simulink model "aircraft_BO_sim"  (R2021b)
settings: Solver=ode45  StartTime=0.0  StopTime=50  RelTol=1e-3  EnableMultiTasking=on
values from neighbouring files (symbols this model uses):
  CD_0 = 0.02    [aircraft_data.m]
  CD_2 = 0.0335    [aircraft_data.m]
  CG = [0 0 0]'    [aircraft_data.m]
  chord = 4.29    [aircraft_data.m]
  CL_0 = 0.11    [aircraft_data.m]
  CL_alpha = 5.5    [aircraft_data.m]
  CL_alphadot = 2.7    [aircraft_data.m]
  Cl_beta = -0.03    [aircraft_data.m]
  Cl_da = -0.07    [aircraft_data.m]
  CL_de = 0.32    [aircraft_data.m]
  Cl_dr = 0.02    [aircraft_data.m]
  CL_dths = -0.32    [aircraft_data.m]
  Cl_p = -0.5    [aircraft_data.m]
  CL_q = 3.3    [aircraft_data.m]
  Cl_r_0 = 0.15    [aircraft_data.m]
  Cl_r_alpha = 0.035    [aircraft_data.m]
  Cm_0 = 0.02    [aircraft_data.m]
  Cm_alpha = -1.5    [aircraft_data.m]
  Cm_alphadot = -12    [aircraft_data.m]
  Cm_de = -1.2    [aircraft_data.m]
  Cm_dths = 1.2    [aircraft_data.m]
  Cm_q = -12    [aircraft_data.m]
  Cn_beta_0 = 0.2    [aircraft_data.m]
  Cn_beta_alpha = -0.0195    [aircraft_data.m]
  Cn_da = -0.03    [aircraft_data.m]
  Cn_dr = -0.09    [aircraft_data.m]
  Cn_p_0 = -0.025    [aircraft_data.m]
  Cn_p_alpha = -0.035    [aircraft_data.m]
  Cn_r = -0.18    [aircraft_data.m]
  CY_beta = -1.42    [aircraft_data.m]
  CY_da = 0.0    (= 0)    [aircraft_data.m]
  CY_dr = 0.05    [aircraft_data.m]
  CY_p = 0.0    (= 0)    [aircraft_data.m]
  CY_r = 0.0    (= 0)    [aircraft_data.m]
  dths_e = x(2)    [trimmed_equations.m]
  em = 1*pi/180    (= 0.0174532925199)    [aircraft_data.m]
  g0 = 9.80665    [aircraft_data.m]
  gamma = 1.4    [aircraft_data.m]
  h0 = 0    [aircraft_data.m]
  h_strat = 20000    [aircraft_data.m]
  h_trop = 11000    [aircraft_data.m]
  Ib = [ Ixx 0   -Ixz ... (first row only)    [aircraft_data.m]
  LEngLoc = [xm -ym zm]'    [aircraft_data.m]
  mass = 57837.5    [aircraft_data.m]
  P0 = 101325    [aircraft_data.m]
  R = 287.0531    [aircraft_data.m]
  REngLoc = [xm  ym zm]'    [aircraft_data.m]
  rho0 = 1.225    [aircraft_data.m]
  T0 = 288.15    [aircraft_data.m]
  Th = -0.0065    [aircraft_data.m]
  wingarea = 122.6    [aircraft_data.m]
  wingspan = 34.10    (= 34.1)    [aircraft_data.m]
undefined symbols (not defined in the file or in its folder): da_e, de_e, dr_e, dth_e, Euler_e, Newton, Omegab_e, Po_e, Raphson, Vb_e
settings Model: Creator=David  LastModifiedBy=dsaussie
settings SolverCC: AlgebraicLoopSolver=TrustRegion
settings DataIOCC: LimitDataPoints=on  SaveFormat=Array  ReturnWorkspaceOutputs=off
settings OptimizationCC: BlockReduction=off  BooleanDataType=off  LifeSpan=inf
settings DebuggingCC: AlgebraicLoopMsg=none  SaveWithParameterizedLinksMsg=none  UnderspecifiedInitializationDetection=Classic  MergeDetectMultiDrivingBlocksExec=none  SignalResolutionControl=TryResolveAllWithWarning  SFUnexpectedBacktrackingDiag=warning  SFNoUnconditionalDefaultTransitionDiag=warning  SFExecutionAtInitializationDiag=none  SFMachineParentedDataDiag=warning  ArithmeticOperatorsInVariantConditions=warning
settings HardwareCC: ProdBitPerPointer=32  ProdBitPerSizeT=32  ProdBitPerPtrDiffT=32  ProdLargestAtomicFloat=None  ProdIntDivRoundTo=Undefined  ProdEndianess=Unspecified  ProdWordSize=32  ProdHWDeviceType=32-bit Generic  TargetUnknown=on
settings ModelReferenceCC: PropagateSignalLabelsOutOfModel=off
settings SFSimCC: SimUseLocalCustomCode=off  CustomCodeUndefinedFunction=UseInterfaceOnly
settings RTWCC: RTWUseLocalCustomCode=off
settings CodeAppCC: StateflowObjectComments=on
settings GRTTargetCC: TargetLangStandard=C89/C90 (ANSI)
settings ConfigComp: CovMetricSettings=dw  CovSaveCumulativeToWorkspaceVar=on  CovSaveSingleToWorkspaceVar=on  CovExternalEMLEnable=off  CovSFcnEnable=off

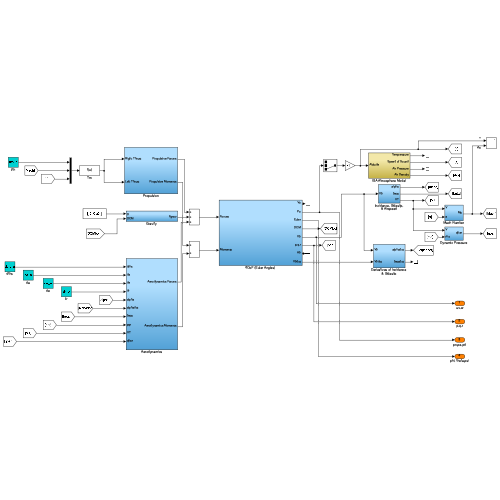
[thumbnail: Simulink's stored preview of the top-level diagram]
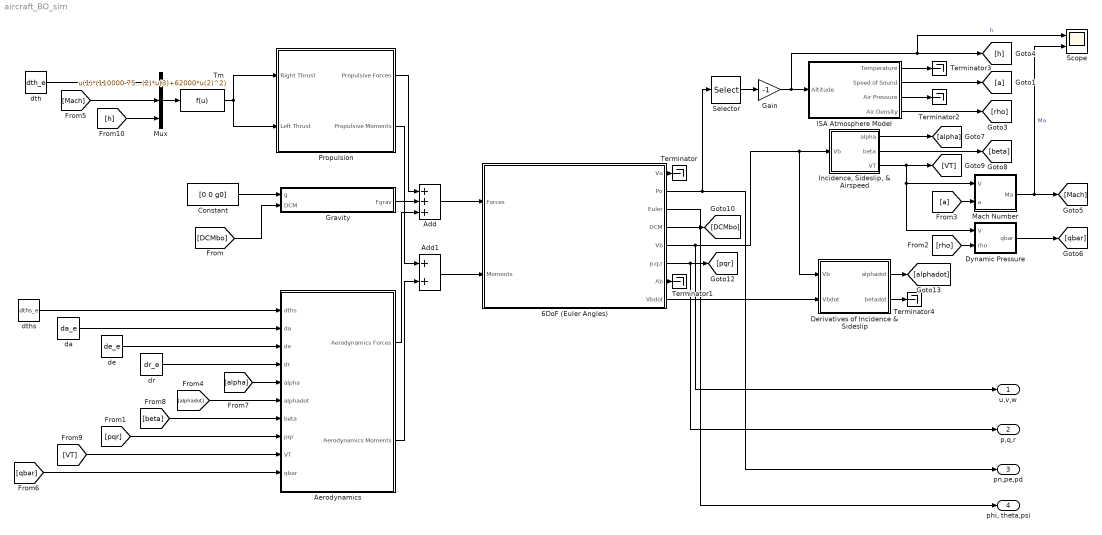
== system aircraft_BO_sim ==
  6DoF (Euler Angles) : Subsystem
  Add : Sum  Inputs=+++
  Add1 : Sum
  Aerodynamics : Subsystem
  Constant : Constant  Value=[0 0 g0]
  Derivatives of Incidence & Sideslip : Subsystem
  Dynamic Pressure : Subsystem
  Gain : Gain  Gain=-1
  "Gravity " : Subsystem
  ISA Atmosphere Model : Subsystem
  "Incidence, Sideslip, & Airspeed" : Subsystem
  Mach Number : Subsystem
  Mux : Mux  Inputs=3
  Propulsion : Subsystem
  Scope : Scope  NumInputPorts=2
  Selector : Selector  InputPortWidth=3  IndexOptions=Index vector (dialog)  Indices=[3]  OutputSizes=1
  Terminator{,1..4} (5 alike) : Terminator
  Tm : Fcn  Expr=u(1)*(110000-75000*u(2)-7.5*u(3)+2*u(2)*u(3)+62000*u(2)^2)
  da : Constant  Value=da_e
  de : Constant  Value=de_e
  dr : Constant  Value=dr_e
  dth : Constant  Value=dth_e
  dths : Constant  Value=dths_e
  u,v,w : Outport
  p,q,r : Outport  Port=2
  pn,pe,pd : Outport  Port=3
  "phi, theta,psi" : Outport  Port=4
  wires:
  Selector/1 -> Gain/1
  ISA Atmosphere Model/1(Temperature) -> Terminator3/1
  ISA Atmosphere Model/2(Speed of Sound) -> [a]
  ISA Atmosphere Model/3(Air Pressure) -> Terminator2/1
  ISA Atmosphere Model/4(Air Density) -> [rho]
  Mach Number/1(Ma) -> Scope/2, [Mach]  "Ma"
  [a] -> Mach Number/2(a)
  [rho] -> Dynamic Pressure/2(rho)
  Dynamic Pressure/1(qbar) -> [qbar]
  "Incidence, Sideslip, & Airspeed"/3(VT) -> Dynamic Pressure/1(V), Mach Number/1(V), [VT]
  "Incidence, Sideslip, & Airspeed"/1(alpha) -> [alpha]
  "Incidence, Sideslip, & Airspeed"/2(beta) -> [beta]
  6DoF (Euler Angles)/4(DCM) -> [DCMbo]
  Propulsion/1(Propulsive Forces) -> Add/1
  Propulsion/2(Propulsive Moments) -> Add1/1
  de/1 -> Aerodynamics/3(de)
  [alpha] -> Aerodynamics/5(alpha)
  [beta] -> Aerodynamics/7(beta)
  [qbar] -> Aerodynamics/10(qbar)
  [VT] -> Aerodynamics/9(VT)
  Aerodynamics/1(Aerodynamics Forces) -> Add/3
  Aerodynamics/2(Aerodynamics Moments) -> Add1/2
  [pqr] -> Aerodynamics/8(pqr)
  [DCMbo] -> "Gravity "/2(DCM)
  Constant/1 -> "Gravity "/1(g)
  "Gravity "/1(Fgrav) -> Add/2
  dth/1 -> Mux/1
  Add/1 -> 6DoF (Euler Angles)/1(Forces)
  Add1/1 -> 6DoF (Euler Angles)/2(Moments)
  6DoF (Euler Angles)/2(Po) -> pn,pe,pd/1, Selector/1
  6DoF (Euler Angles)/3(Euler) -> "phi, theta,psi"/1
  6DoF (Euler Angles)/6(p,q,r) -> p,q,r/1, [pqr]
  6DoF (Euler Angles)/5(Vb) -> u,v,w/1, Derivatives of Incidence & Sideslip/1(Vb), "Incidence, Sideslip, & Airspeed"/1(Vb)
  dr/1 -> Aerodynamics/4(dr)
  da/1 -> Aerodynamics/2(da)
  6DoF (Euler Angles)/8(Vbdot) -> Derivatives of Incidence & Sideslip/2(Vbdot)
  Derivatives of Incidence & Sideslip/1(alphadot) -> [alphadot]
  Derivatives of Incidence & Sideslip/2(betadot) -> Terminator4/1
  [alphadot] -> Aerodynamics/6(alphadot)
  Mux/1 -> Tm/1
  6DoF (Euler Angles)/1(Vo) -> Terminator/1
  6DoF (Euler Angles)/7(Ab) -> Terminator1/1
  Gain/1 -> ISA Atmosphere Model/1(Altitude), Scope/1, [h]  "h"
  [Mach] -> Mux/2
  [h] -> Mux/3
  Tm/1 -> Propulsion/1(Right Thrust), Propulsion/2(Left Thrust)
  dths/1 -> Aerodynamics/1(dths)

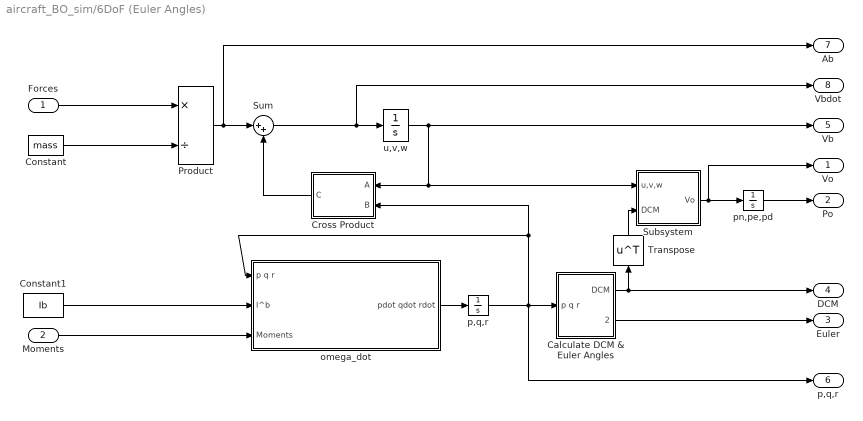
== system aircraft_BO_sim/6DoF (Euler Angles) ==
  Forces : Inport
  Moments : Inport  Port=2
  "Calculate DCM & Euler Angles " : Subsystem
  Constant : Constant  Value=mass  OutDataTypeStr=Inherit: Inherit via back propagation
  Constant1 : Constant  Value=Ib  OutDataTypeStr=Inherit: Inherit via back propagation
  Cross Product : Subsystem
  Product : Product  Inputs=*/  SaturateOnIntegerOverflow=on  OutDataTypeStr=Inherit: Same as first input
  Subsystem : Subsystem
  Sum : Sum  Inputs=|++  SaturateOnIntegerOverflow=on
  Transpose : Math  Operator=transpose  SignedPower=on  SaturateOnIntegerOverflow=on
  omega_dot : Subsystem
  "p,q,r " : Integrator  InitialCondition=Omegab_e
  pn,pe,pd : Integrator  InitialCondition=Po_e
  u,v,w : Integrator  InitialCondition=Vb_e
  Vo : Outport
  Po : Outport  Port=2
  Euler : Outport  Port=3
  DCM : Outport  Port=4
  Vb : Outport  Port=5
  p,q,r : Outport  Port=6
  Ab : Outport  Port=7
  Vbdot : Outport  Port=8
  wires:
  Moments/1 -> omega_dot/3(Moments)
  "p,q,r "/1 -> Cross Product/2(B), omega_dot/1(p q r), p,q,r/1, "Calculate DCM & Euler Angles "/1("p q r ")
  Sum/1 -> Vbdot/1, u,v,w/1
  u,v,w/1 -> Vb/1, Cross Product/1(A), Subsystem/1(u,v,w)
  Subsystem/1(Vo) -> Vo/1, pn,pe,pd/1
  pn,pe,pd/1 -> Po/1
  Forces/1 -> Product/1
  Constant/1 -> Product/2
  Transpose/1 -> Subsystem/2(DCM)
  "Calculate DCM & Euler Angles "/1("DCM ") -> DCM/1, Transpose/1
  Product/1 -> Ab/1, Sum/1
  Cross Product/1(C) -> Sum/2
  "Calculate DCM & Euler Angles "/2(Euler) -> Euler/1
  Constant1/1 -> omega_dot/2(I^b)
  omega_dot/1(pdot qdot rdot) -> "p,q,r "/1

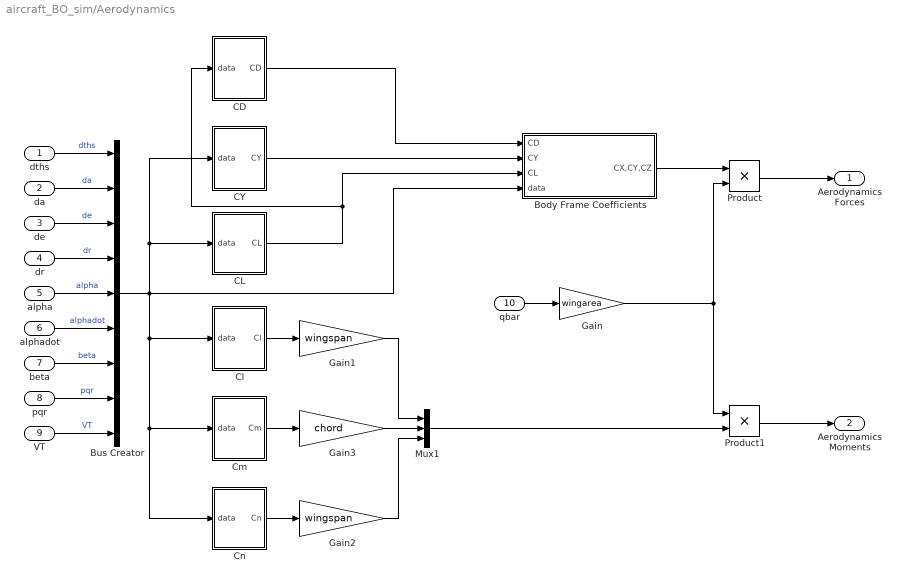
== system aircraft_BO_sim/Aerodynamics ==
  dths : Inport
  da : Inport  Port=2
  de : Inport  Port=3
  dr : Inport  Port=4
  alpha : Inport  Port=5
  alphadot : Inport  Port=6
  beta : Inport  Port=7
  pqr : Inport  Port=8
  VT : Inport  Port=9
  qbar : Inport  Port=10
  Body Frame Coefficients : Subsystem
  Bus Creator : BusCreator  Inputs=9
  CD : Subsystem
  CL : Subsystem
  CY : Subsystem
  Cl : Subsystem
  Cm : Subsystem
  Cn : Subsystem
  Gain : Gain  Gain=wingarea
  Gain1 : Gain  Gain=wingspan
  Gain2 : Gain  Gain=wingspan
  Gain3 : Gain  Gain=chord
  Mux1 : Mux  Inputs=3
  Product : Product  RndMeth=Zero
  Product1 : Product  RndMeth=Zero
  Aerodynamics Forces : Outport
  Aerodynamics Moments : Outport  Port=2
  wires:
  de/1 -> Bus Creator/3  "de"
  da/1 -> Bus Creator/2  "da"
  dr/1 -> Bus Creator/4  "dr"
  alpha/1 -> Bus Creator/5  "alpha"
  beta/1 -> Bus Creator/7  "beta"
  pqr/1 -> Bus Creator/8  "pqr"
  Bus Creator/1 -> Body Frame Coefficients/4(data), Cn/1(data), Cm/1(data), Cl/1(data), CY/1(data), CL/1(data)
  CL/1(CL) -> CD/1(data), Body Frame Coefficients/3(CL)
  Cl/1(Cl) -> Gain1/1
  Cm/1(Cm) -> Gain3/1
  Cn/1(Cn) -> Gain2/1
  VT/1 -> Bus Creator/9  "VT"
  qbar/1 -> Gain/1
  Gain/1 -> Product/2, Product1/1
  Mux1/1 -> Product1/2
  Gain1/1 -> Mux1/1
  Gain2/1 -> Mux1/3
  Gain3/1 -> Mux1/2
  Product/1 -> Aerodynamics Forces/1
  Product1/1 -> Aerodynamics Moments/1
  CD/1(CD) -> Body Frame Coefficients/1(CD)
  CY/1(CY) -> Body Frame Coefficients/2(CY)
  Body Frame Coefficients/1(CX,CY,CZ) -> Product/1
  alphadot/1 -> Bus Creator/6  "alphadot"
  dths/1 -> Bus Creator/1  "dths"

== system aircraft_BO_sim/Derivatives of Incidence & Sideslip ==
  Vb : Inport
  Vbdot : Inport  Port=2
  Airspeed : Sqrt  AlgorithmType=Newton-Raphson  SaturateOnIntegerOverflow=on
  Fcn : Fcn  Expr=(u(1)*u(6)-u(3)*u(4))/(u(1)^2+u(3)^2)
  Fcn1 : Fcn  Expr=(u(5)*u(7)-u(8)*u(2))/sqrt(u(1)^2+u(3)^2)/u(7)
  Mux : Mux  Inputs=3
  Mux1 : Mux
  VTdot : Fcn  Expr=(u(2)*u(5)+u(3)*u(6)+u(4)*u(7))/u(1)
  dot : Subsystem
  alphadot : Outport
  betadot : Outport  Port=2
  wires:
  Mux1/1 -> Fcn1/1, Fcn/1
  Vb/1 -> Mux1/1, Mux/2, dot/1(In1)
  Vbdot/1 -> Mux1/2, Mux/3
  Fcn/1 -> alphadot/1
  Fcn1/1 -> betadot/1
  dot/1(Out1) -> Airspeed/1
  Airspeed/1 -> Mux1/3, Mux/1
  Mux/1 -> VTdot/1
  VTdot/1 -> Mux1/4

== system aircraft_BO_sim/Dynamic Pressure ==
  V : Inport
  rho : Inport  Port=2
  1/2rhoV^2 : Gain  Gain=1/2  SaturateOnIntegerOverflow=on  OutDataTypeStr=Inherit: Same as input  ParamDataTypeStr=Inherit: Same as input
  Product2 : Product  Inputs=3  InputSameDT=on  SaturateOnIntegerOverflow=on  OutDataTypeStr=Inherit: Same as first input
  qbar : Outport
  wires:
  1/2rhoV^2/1 -> qbar/1
  Product2/1 -> 1/2rhoV^2/1
  rho/1 -> Product2/3
  V/1 -> Product2/2, Product2/1

== system aircraft_BO_sim/Gravity  ==
  g : Inport
  DCM : Inport  Port=2
  Gravity in Earth Axes : Gain  Gain=mass  SaturateOnIntegerOverflow=on  OutDataTypeStr=Inherit: Same as input  ParamDataTypeStr=Inherit: Same as input
  Inertial to Body : Product  Multiplication=Matrix(*)  InputSameDT=on  SaturateOnIntegerOverflow=on  OutDataTypeStr=Inherit: Same as first input
  Reshape : Reshape  OutputDimensionality=Column vector (2-D)
  Reshape1 : Reshape
  Fgrav : Outport
  wires:
  Inertial to Body/1 -> Reshape1/1
  g/1 -> Gravity in Earth Axes/1
  DCM/1 -> Inertial to Body/1
  Gravity in Earth Axes/1 -> Reshape/1
  Reshape/1 -> Inertial to Body/2
  Reshape1/1 -> Fgrav/1

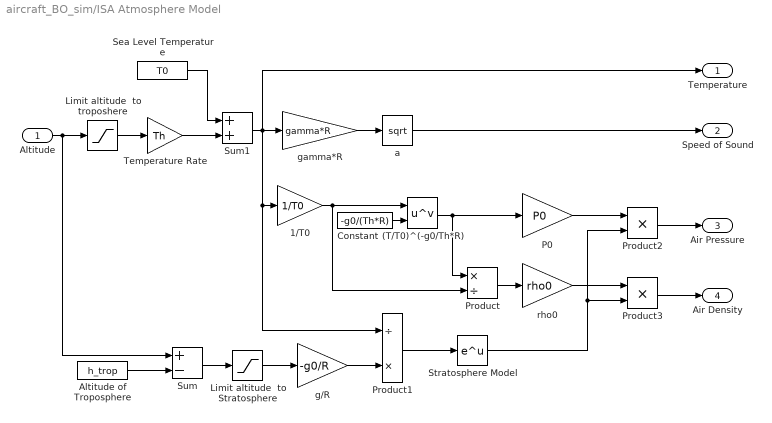
== system aircraft_BO_sim/ISA Atmosphere Model ==
  Altitude : Inport
  "(T/T0)^(-g0/Th*R) " : Math  Operator=pow  SignedPower=on  SaturateOnIntegerOverflow=on
  1/T0 : Gain  Gain=1/T0  SaturateOnIntegerOverflow=on  OutDataTypeStr=Inherit: Same as input  ParamDataTypeStr=Inherit: Same as input
  Altitude of Troposphere : Constant  Value=h_trop  OutDataTypeStr=Inherit: Inherit via back propagation
  Constant : Constant  Value=-g0/(Th*R)  OutDataTypeStr=Inherit: Inherit via back propagation
  Limit altitude  to Stratosphere : Saturate  UpperLimit=h_strat-h_trop  LowerLimit=0
  Limit altitude  to troposhere : Saturate  UpperLimit=h_trop  LowerLimit=h0
  P0 : Gain  Gain=P0  SaturateOnIntegerOverflow=on  OutDataTypeStr=Inherit: Same as input  ParamDataTypeStr=Inherit: Same as input
  Product : Product  Inputs=*/  InputSameDT=on  SaturateOnIntegerOverflow=on  OutDataTypeStr=Inherit: Same as first input
  Product1 : Product  Inputs=/*  InputSameDT=on  SaturateOnIntegerOverflow=on  OutDataTypeStr=Inherit: Same as first input
  Product2 : Product  InputSameDT=on  SaturateOnIntegerOverflow=on  OutDataTypeStr=Inherit: Same as first input
  Product3 : Product  InputSameDT=on  SaturateOnIntegerOverflow=on  OutDataTypeStr=Inherit: Same as first input
  Sea Level Temperature : Constant  Value=T0  OutDataTypeStr=Inherit: Inherit via back propagation
  Stratosphere Model : Math  SignedPower=on  SaturateOnIntegerOverflow=on
  Sum : Sum  Inputs=+-  InputSameDT=on  SaturateOnIntegerOverflow=on  OutDataTypeStr=Inherit: Same as first input
  Sum1 : Sum  InputSameDT=on  SaturateOnIntegerOverflow=on  OutDataTypeStr=Inherit: Same as first input
  Temperature Rate : Gain  Gain=Th  SaturateOnIntegerOverflow=on  OutDataTypeStr=Inherit: Same as input  ParamDataTypeStr=Inherit: Same as input
  a : Sqrt  AlgorithmType=Newton-Raphson  SaturateOnIntegerOverflow=on
  g/R : Gain  Gain=-g0/R  SaturateOnIntegerOverflow=on  OutDataTypeStr=Inherit: Same as input  ParamDataTypeStr=Inherit: Same as input
  gamma*R : Gain  Gain=gamma*R  SaturateOnIntegerOverflow=on  OutDataTypeStr=Inherit: Same as input  ParamDataTypeStr=Inherit: Same as input
  rho0 : Gain  Gain=rho0  SaturateOnIntegerOverflow=on  OutDataTypeStr=Inherit: Same as input  ParamDataTypeStr=Inherit: Same as input
  Temperature : Outport
  Speed of Sound : Outport  Port=2
  Air Pressure : Outport  Port=3
  Air Density : Outport  Port=4
  wires:
  1/T0/1 -> "(T/T0)^(-g0/Th*R) "/1, Product/2
  gamma*R/1 -> a/1
  a/1 -> Speed of Sound/1
  Sum1/1 -> Temperature/1, gamma*R/1, 1/T0/1, Product1/1
  Sum/1 -> Limit altitude  to Stratosphere/1
  Product2/1 -> Air Pressure/1
  rho0/1 -> Product3/1
  Product3/1 -> Air Density/1
  Stratosphere Model/1 -> Product2/2, Product3/2
  Sea Level Temperature/1 -> Sum1/1
  P0/1 -> Product2/1
  Constant/1 -> "(T/T0)^(-g0/Th*R) "/2
  Altitude/1 -> Sum/1, Limit altitude  to troposhere/1
  Limit altitude  to troposhere/1 -> Temperature Rate/1
  Product/1 -> rho0/1
  "(T/T0)^(-g0/Th*R) "/1 -> Product/1, P0/1
  Temperature Rate/1 -> Sum1/2
  g/R/1 -> Product1/2
  Product1/1 -> Stratosphere Model/1
  Altitude of Troposphere/1 -> Sum/2
  Limit altitude  to Stratosphere/1 -> g/R/1

== system aircraft_BO_sim/Incidence, Sideslip, & Airspeed ==
  Vb : Inport
  Airspeed : Sqrt  AlgorithmType=Newton-Raphson  SaturateOnIntegerOverflow=on
  Demux1 : Demux  Outputs=3
      settings: DisplayOption=none
  Incidence : Trigonometry  Operator=atan2
  Product : Product  Inputs=*/  SaturateOnIntegerOverflow=on  OutDataTypeStr=Inherit: Same as first input
  Sideslip : Trigonometry  Operator=asin
  dot : Subsystem
  alpha : Outport  InitialOutput=0
  beta : Outport  Port=2  InitialOutput=0
  VT : Outport  Port=3  InitialOutput=0
  wires:
  Product/1 -> Sideslip/1
  Demux1/1 -> Incidence/2
  Demux1/3 -> Incidence/1
  dot/1(Out1) -> Airspeed/1
  Airspeed/1 -> VT/1, Product/2
  Incidence/1 -> alpha/1
  Vb/1 -> dot/1(In1), Demux1/1
  Sideslip/1 -> beta/1
  Demux1/2 -> Product/1

== system aircraft_BO_sim/Mach Number ==
  V : Inport
  a : Inport  Port=2
  Product1 : Product  Inputs=*/  InputSameDT=on  SaturateOnIntegerOverflow=on  OutDataTypeStr=Inherit: Same as first input
  Ma : Outport
  wires:
  Product1/1 -> Ma/1
  V/1 -> Product1/1
  a/1 -> Product1/2

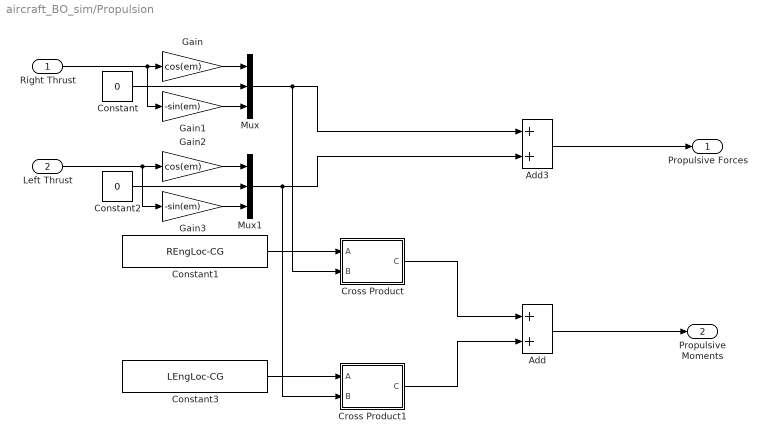
== system aircraft_BO_sim/Propulsion ==
  Right Thrust : Inport
  Left Thrust : Inport  Port=2
  Add : Sum
  Add3 : Sum
  Constant : Constant  Value=0
  Constant1 : Constant  Value=REngLoc-CG
  Constant2 : Constant  Value=0
  Constant3 : Constant  Value=LEngLoc-CG
  Cross Product : Subsystem
  Cross Product1 : Subsystem
  Gain : Gain  Gain=cos(em)
  Gain1 : Gain  Gain=-sin(em)
  Gain2 : Gain  Gain=cos(em)
  Gain3 : Gain  Gain=-sin(em)
  Mux : Mux  Inputs=3
  Mux1 : Mux  Inputs=3
  Propulsive Forces : Outport
  Propulsive Moments : Outport  Port=2
  wires:
  Constant/1 -> Mux/2
  Right Thrust/1 -> Gain1/1, Gain/1
  Add/1 -> Propulsive Moments/1
  Cross Product/1(C) -> Add/1
  Cross Product1/1(C) -> Add/2
  Mux1/1 -> Cross Product1/2(B), Add3/2
  Add3/1 -> Propulsive Forces/1
  Mux/1 -> Cross Product/2(B), Add3/1
  Constant1/1 -> Cross Product/1(A)
  Constant3/1 -> Cross Product1/1(A)
  Gain/1 -> Mux/1
  Gain1/1 -> Mux/3
  Constant2/1 -> Mux1/2
  Left Thrust/1 -> Gain3/1, Gain2/1
  Gain2/1 -> Mux1/1
  Gain3/1 -> Mux1/3

== system aircraft_BO_sim/6DoF (Euler Angles)/Calculate DCM & Euler Angles  ==
  "p q r " : Inport
  DCM : Subsystem
  Selector : Selector  InputPortWidth=3  IndexOptions=Index vector (dialog)  Indices=[3 2 1]  OutputSizes=1
  Subsystem : Subsystem
  phi theta psi : Integrator  InitialCondition=Euler_e
  "DCM " : Outport
  Euler : Outport  Port=2
  wires:
  Selector/1 -> DCM/1(Psi,Theta,Phi)
  phi theta psi/1 -> Subsystem/2(phi theta psi), Euler/1, Selector/1
  Subsystem/1(phidot thetadot psidot) -> phi theta psi/1
  "p q r "/1 -> Subsystem/1(p q r)
  DCM/1(DCM) -> "DCM "/1

== system aircraft_BO_sim/6DoF (Euler Angles)/Cross Product ==
  A : Inport
  B : Inport  Port=2
  Subsystem : Subsystem
  Subsystem2 : Subsystem
  Sum1 : Sum  Inputs=+|-  InputSameDT=on  SaturateOnIntegerOverflow=on  OutDataTypeStr=Inherit: Same as first input
  C : Outport
  wires:
  A/1 -> Subsystem/1(A), Subsystem2/1(A)
  Subsystem2/1(Out1) -> Sum1/1
  Subsystem/1(Out1) -> Sum1/2
  Sum1/1 -> C/1
  B/1 -> Subsystem/2(B), Subsystem2/2(B)

== system aircraft_BO_sim/6DoF (Euler Angles)/Subsystem ==
  u,v,w : Inport
  DCM : Inport  Port=2
  Product1 : Product  Multiplication=Matrix(*)  InputSameDT=on  SaturateOnIntegerOverflow=on  OutDataTypeStr=Inherit: Same as first input
  Reshape1 : Reshape  OutputDimensionality=Column vector (2-D)
  Reshape2 : Reshape
  Vo : Outport
  wires:
  Reshape2/1 -> Vo/1
  Reshape1/1 -> Product1/2
  u,v,w/1 -> Reshape1/1
  DCM/1 -> Product1/1
  Product1/1 -> Reshape2/1

== system aircraft_BO_sim/6DoF (Euler Angles)/omega_dot ==
  p q r : Inport
  I^b : Inport  Port=2
  Moments : Inport  Port=3
  Cross Product : Subsystem
  Product2 : Product  Inputs=*/  Multiplication=Matrix(*)  SaturateOnIntegerOverflow=on  OutDataTypeStr=Inherit: Same as first input
  Reshape : Reshape
  Reshape1 : Reshape  OutputDimensionality=Row vector (2-D)
  Selector : Selector  NumberOfDimensions=2  InputPortWidth=2  IndexOptions=Index vector (dialog),Select all  Indices=1:3,-1  OutputSizes=1
  Selector2 : Selector  NumberOfDimensions=2  InputPortWidth=2  IndexOptions=Index vector (dialog),Select all  Indices=1:3,-1  OutputSizes=1
  Subsystem1 : Subsystem
  Sum2 : Sum  Inputs=|+-  SaturateOnIntegerOverflow=on
  pdot qdot rdot : Outport
  wires:
  I^b/1 -> Selector2/1, Selector/1
  Selector2/1 -> Product2/2
  Selector/1 -> Subsystem1/2(Inertia)
  Reshape/1 -> pdot qdot rdot/1
  Moments/1 -> Sum2/1
  Sum2/1 -> Reshape1/1
  Product2/1 -> Reshape/1
  p q r/1 -> Cross Product/1(A), Subsystem1/1(p q r)
  Reshape1/1 -> Product2/1
  Subsystem1/1(I * w) -> Cross Product/2(B)
  Cross Product/1(C) -> Sum2/2

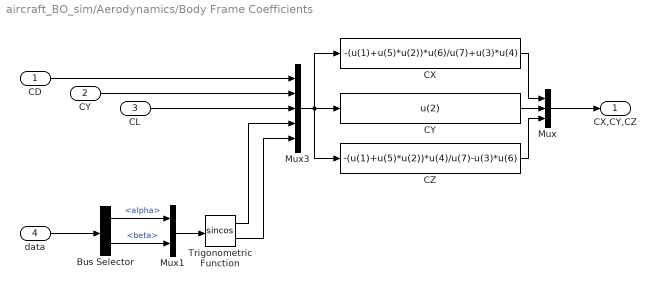
== system aircraft_BO_sim/Aerodynamics/Body Frame Coefficients ==
  CD : Inport
  CY : Inport  Port=2
  CL : Inport  Port=3
  data : Inport  Port=4
  " CY" : Fcn  Expr=u(2)
  Bus Selector : BusSelector  OutputSignals=alpha,beta
  CX : Fcn  Expr=-(u(1)+u(5)*u(2))*u(6)/u(7)+u(3)*u(4)
  CZ : Fcn  Expr=-(u(1)+u(5)*u(2))*u(4)/u(7)-u(3)*u(6)
  Mux : Mux  Inputs=3
  Mux1 : Mux  Inputs=2
  Mux3 : Mux  Inputs=5
  Trigonometric Function : Trigonometry  Operator=sincos
  CX,CY,CZ : Outport
  wires:
  CD/1 -> Mux3/1
  Mux/1 -> CX,CY,CZ/1
  CY/1 -> Mux3/2
  Trigonometric Function/1 -> Mux3/4
  Trigonometric Function/2 -> Mux3/5
  CL/1 -> Mux3/3
  data/1 -> Bus Selector/1
  Bus Selector/1 -> Mux1/1  "<alpha>"
  Bus Selector/2 -> Mux1/2  "<beta>"
  Mux1/1 -> Trigonometric Function/1
  Mux3/1 -> CX/1, " CY"/1, CZ/1
  " CY"/1 -> Mux/2
  CX/1 -> Mux/1
  CZ/1 -> Mux/3

== system aircraft_BO_sim/Aerodynamics/CD ==
  data : Inport
  Add : Sum
  Constant : Constant  Value=CD_0
  Gain1 : Gain  Gain=CD_2
  Product : Product
  CD : Outport
  wires:
  Constant/1 -> Add/1
  Add/1 -> CD/1
  data/1 -> Product/2, Product/1
  Product/1 -> Gain1/1
  Gain1/1 -> Add/2

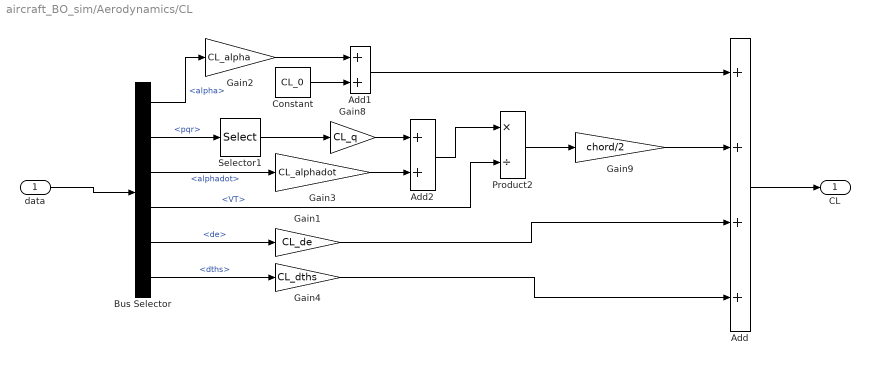
== system aircraft_BO_sim/Aerodynamics/CL ==
  data : Inport
  Add : Sum  Inputs=++++
  Add1 : Sum
  Add2 : Sum
  Bus Selector : BusSelector  OutputSignals=alpha,pqr,alphadot,VT,de,dths
  Constant : Constant  Value=CL_0
  Gain1 : Gain  Gain=CL_de
  Gain2 : Gain  Gain=CL_alpha
  Gain3 : Gain  Gain=CL_alphadot
  Gain4 : Gain  Gain=CL_dths
  Gain8 : Gain  Gain=CL_q
  Gain9 : Gain  Gain=chord/2
  Product2 : Product  Inputs=*/  RndMeth=Zero
  Selector1 : Selector  InputPortWidth=3  IndexOptions=Index vector (dialog)  Indices=2  OutputSizes=1
  CL : Outport
  wires:
  Add/1 -> CL/1
  data/1 -> Bus Selector/1
  Bus Selector/1 -> Gain2/1  "<alpha>"
  Bus Selector/5 -> Gain1/1  "<de>"
  Constant/1 -> Add1/2
  Add1/1 -> Add/1
  Bus Selector/3 -> Gain3/1  "<alphadot>"
  Gain3/1 -> Add2/2
  Bus Selector/2 -> Selector1/1  "<pqr>"
  Selector1/1 -> Gain8/1
  Product2/1 -> Gain9/1
  Bus Selector/4 -> Product2/2  "<VT>"
  Gain8/1 -> Add2/1
  Gain9/1 -> Add/2
  Gain1/1 -> Add/3
  Add2/1 -> Product2/1
  Bus Selector/6 -> Gain4/1  "<dths>"
  Gain4/1 -> Add/4
  Gain2/1 -> Add1/1

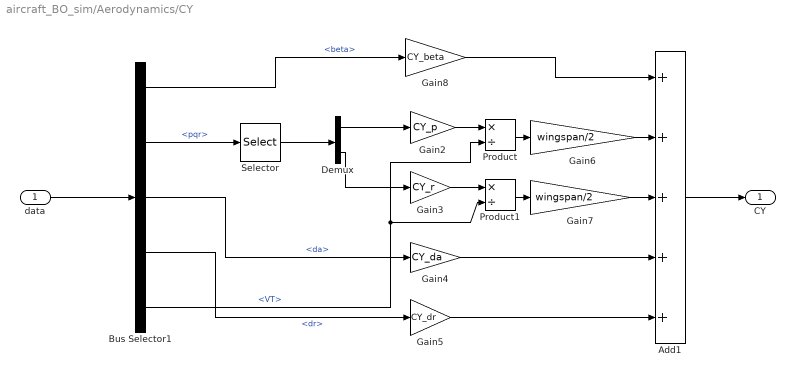
== system aircraft_BO_sim/Aerodynamics/CY ==
  data : Inport
  Add1 : Sum  Inputs=+++++
  Bus Selector1 : BusSelector  OutputSignals=beta,pqr,da,dr,VT
  Demux : Demux  Outputs=2
  Gain2 : Gain  Gain=CY_p
  Gain3 : Gain  Gain=CY_r
  Gain4 : Gain  Gain=CY_da
  Gain5 : Gain  Gain=CY_dr
  Gain6 : Gain  Gain=wingspan/2
  Gain7 : Gain  Gain=wingspan/2
  Gain8 : Gain  Gain=CY_beta
  Product : Product  Inputs=*/  RndMeth=Zero
  Product1 : Product  Inputs=*/  RndMeth=Zero
  Selector : Selector  InputPortWidth=3  IndexOptions=Index vector (dialog)  Indices=[1 3]  OutputSizes=1
  CY : Outport
  wires:
  data/1 -> Bus Selector1/1
  Add1/1 -> CY/1
  Gain8/1 -> Add1/1
  Bus Selector1/1 -> Gain8/1  "<beta>"
  Bus Selector1/2 -> Selector/1  "<pqr>"
  Bus Selector1/3 -> Gain4/1  "<da>"
  Bus Selector1/4 -> Gain5/1  "<dr>"
  Selector/1 -> Demux/1
  Demux/1 -> Gain2/1
  Demux/2 -> Gain3/1
  Gain4/1 -> Add1/4
  Gain5/1 -> Add1/5
  Product/1 -> Gain6/1
  Gain2/1 -> Product/1
  Product1/1 -> Gain7/1
  Gain3/1 -> Product1/1
  Bus Selector1/5 -> Product/2, Product1/2  "<VT>"
  Gain6/1 -> Add1/2
  Gain7/1 -> Add1/3

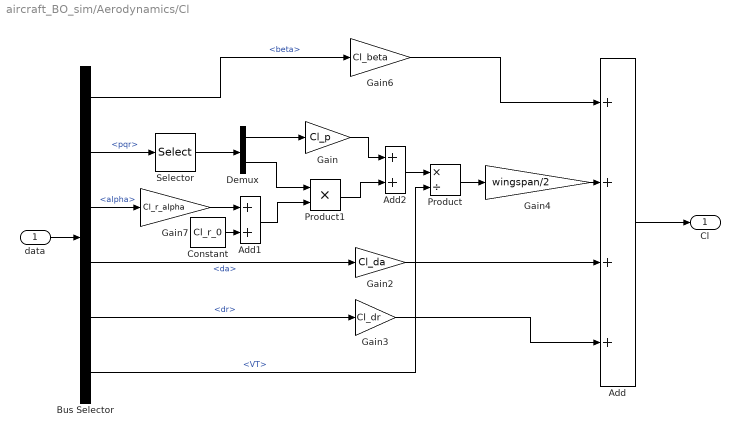
== system aircraft_BO_sim/Aerodynamics/Cl ==
  data : Inport
  Add : Sum  Inputs=++++
  Add1 : Sum
  Add2 : Sum
  Bus Selector : BusSelector  OutputSignals=beta,pqr,alpha,da,dr,VT
  Constant : Constant  Value=Cl_r_0
  Demux : Demux  Outputs=2
  Gain : Gain  Gain=Cl_p
  Gain2 : Gain  Gain=Cl_da
  Gain3 : Gain  Gain=Cl_dr
  Gain4 : Gain  Gain=wingspan/2
  Gain6 : Gain  Gain=Cl_beta
  Gain7 : Gain  Gain=Cl_r_alpha
  Product : Product  Inputs=*/  RndMeth=Zero
  Product1 : Product  Inputs=**  RndMeth=Zero
  Selector : Selector  InputPortWidth=3  IndexOptions=Index vector (dialog)  Indices=[1 3]  OutputSizes=1
  Cl : Outport
  wires:
  data/1 -> Bus Selector/1
  Add/1 -> Cl/1
  Gain6/1 -> Add/1
  Bus Selector/1 -> Gain6/1  "<beta>"
  Bus Selector/2 -> Selector/1  "<pqr>"
  Bus Selector/4 -> Gain2/1  "<da>"
  Bus Selector/5 -> Gain3/1  "<dr>"
  Selector/1 -> Demux/1
  Demux/1 -> Gain/1
  Demux/2 -> Product1/1
  Gain2/1 -> Add/3
  Gain3/1 -> Add/4
  Product/1 -> Gain4/1
  Gain/1 -> Add2/1
  Bus Selector/6 -> Product/2  "<VT>"
  Gain4/1 -> Add/2
  Bus Selector/3 -> Gain7/1  "<alpha>"
  Add1/1 -> Product1/2
  Constant/1 -> Add1/2
  Gain7/1 -> Add1/1
  Add2/1 -> Product/1
  Product1/1 -> Add2/2

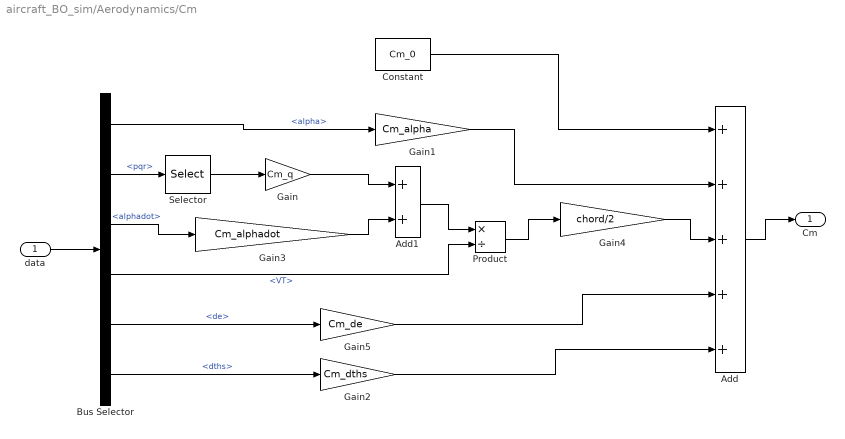
== system aircraft_BO_sim/Aerodynamics/Cm ==
  data : Inport
  Add : Sum  Inputs=+++++
  Add1 : Sum
  Bus Selector : BusSelector  OutputSignals=alpha,pqr,alphadot,VT,de,dths
  Constant : Constant  Value=Cm_0
  Gain : Gain  Gain=Cm_q
  Gain1 : Gain  Gain=Cm_alpha
  Gain2 : Gain  Gain=Cm_dths
  Gain3 : Gain  Gain=Cm_alphadot
  Gain4 : Gain  Gain=chord/2
  Gain5 : Gain  Gain=Cm_de
  Product : Product  Inputs=*/  RndMeth=Zero
  Selector : Selector  InputPortWidth=3  IndexOptions=Index vector (dialog)  Indices=[2]  OutputSizes=1
  Cm : Outport
  wires:
  data/1 -> Bus Selector/1
  Add/1 -> Cm/1
  Constant/1 -> Add/1
  Bus Selector/2 -> Selector/1  "<pqr>"
  Selector/1 -> Gain/1
  Product/1 -> Gain4/1
  Gain/1 -> Add1/1
  Gain4/1 -> Add/3
  Bus Selector/1 -> Gain1/1  "<alpha>"
  Bus Selector/5 -> Gain5/1  "<de>"
  Bus Selector/4 -> Product/2  "<VT>"
  Gain1/1 -> Add/2
  Gain5/1 -> Add/4
  Bus Selector/3 -> Gain3/1  "<alphadot>"
  Gain3/1 -> Add1/2
  Add1/1 -> Product/1
  Bus Selector/6 -> Gain2/1  "<dths>"
  Gain2/1 -> Add/5

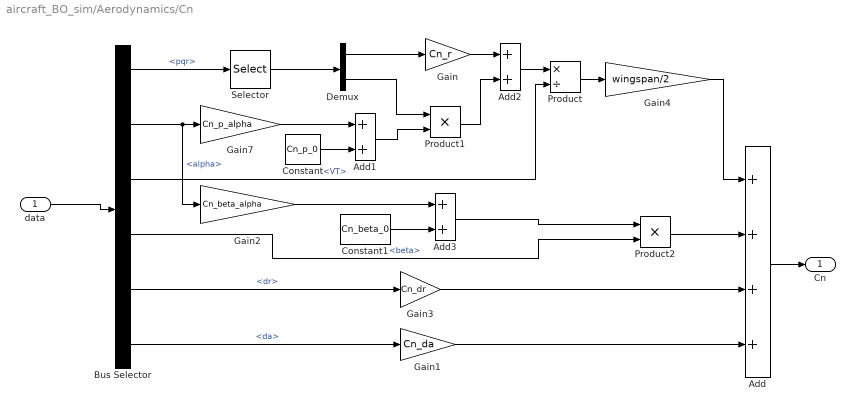
== system aircraft_BO_sim/Aerodynamics/Cn ==
  data : Inport
  Add : Sum  Inputs=++++
  Add1 : Sum
  Add2 : Sum
  Add3 : Sum
  Bus Selector : BusSelector  OutputSignals=pqr,alpha,VT,beta,dr,da
  Constant : Constant  Value=Cn_p_0
  Constant1 : Constant  Value=Cn_beta_0
  Demux : Demux  Outputs=2
  Gain : Gain  Gain=Cn_r
  Gain1 : Gain  Gain=Cn_da
  Gain2 : Gain  Gain=Cn_beta_alpha
  Gain3 : Gain  Gain=Cn_dr
  Gain4 : Gain  Gain=wingspan/2
  Gain7 : Gain  Gain=Cn_p_alpha
  Product : Product  Inputs=*/  RndMeth=Zero
  Product1 : Product  Inputs=**  RndMeth=Zero
  Product2 : Product  Inputs=**  RndMeth=Zero
  Selector : Selector  InputPortWidth=3  IndexOptions=Index vector (dialog)  Indices=[3 1]  OutputSizes=1
  Cn : Outport
  wires:
  data/1 -> Bus Selector/1
  Add/1 -> Cn/1
  Bus Selector/5 -> Gain3/1  "<dr>"
  Gain3/1 -> Add/3
  Bus Selector/3 -> Product/2  "<VT>"
  Product2/1 -> Add/2
  Gain4/1 -> Add/1
  Bus Selector/6 -> Gain1/1  "<da>"
  Gain1/1 -> Add/4
  Selector/1 -> Demux/1
  Demux/1 -> Gain/1
  Demux/2 -> Product1/1
  Product/1 -> Gain4/1
  Gain/1 -> Add2/1
  Bus Selector/4 -> Product2/2  "<beta>"
  Bus Selector/2 -> Gain2/1, Gain7/1  "<alpha>"
  Add1/1 -> Product1/2
  Constant/1 -> Add1/2
  Gain7/1 -> Add1/1
  Add2/1 -> Product/1
  Product1/1 -> Add2/2
  Bus Selector/1 -> Selector/1  "<pqr>"
  Constant1/1 -> Add3/2
  Add3/1 -> Product2/1
  Gain2/1 -> Add3/1

== system aircraft_BO_sim/Derivatives of Incidence & Sideslip/dot ==
  In1 : Inport
  Demux2 : Demux  Outputs=3
  Product1 : Product  RndMeth=Zero
  Product2 : Product  RndMeth=Zero
  Product3 : Product  RndMeth=Zero
  Sum : Sum  Inputs=+++
  Out1 : Outport
  wires:
  Product1/1 -> Sum/1
  Demux2/3 -> Product3/2, Product3/1
  Product2/1 -> Sum/2
  Sum/1 -> Out1/1
  In1/1 -> Demux2/1
  Demux2/2 -> Product2/1, Product2/2
  Product3/1 -> Sum/3
  Demux2/1 -> Product1/2, Product1/1

== system aircraft_BO_sim/Incidence, Sideslip, & Airspeed/dot ==
  In1 : Inport
  Demux2 : Demux  Outputs=3
  Product1 : Product  RndMeth=Zero
  Product2 : Product  RndMeth=Zero
  Product3 : Product  RndMeth=Zero
  Sum : Sum  Inputs=+++
  Out1 : Outport
  wires:
  Product1/1 -> Sum/1
  Demux2/3 -> Product3/2, Product3/1
  Product2/1 -> Sum/2
  Sum/1 -> Out1/1
  In1/1 -> Demux2/1
  Demux2/2 -> Product2/1, Product2/2
  Product3/1 -> Sum/3
  Demux2/1 -> Product1/2, Product1/1

== system aircraft_BO_sim/Propulsion/Cross Product ==
  A : Inport
  B : Inport  Port=2
  Subsystem : Subsystem
  Subsystem2 : Subsystem
  Sum1 : Sum  Inputs=+|-  InputSameDT=on  SaturateOnIntegerOverflow=on  OutDataTypeStr=Inherit: Same as first input
  C : Outport
  wires:
  A/1 -> Subsystem/1(A), Subsystem2/1(A)
  Subsystem2/1(Out1) -> Sum1/1
  Subsystem/1(Out1) -> Sum1/2
  Sum1/1 -> C/1
  B/1 -> Subsystem/2(B), Subsystem2/2(B)

== system aircraft_BO_sim/Propulsion/Cross Product1 ==
  A : Inport
  B : Inport  Port=2
  Subsystem : Subsystem
  Subsystem2 : Subsystem
  Sum1 : Sum  Inputs=+|-  InputSameDT=on  SaturateOnIntegerOverflow=on  OutDataTypeStr=Inherit: Same as first input
  C : Outport
  wires:
  A/1 -> Subsystem/1(A), Subsystem2/1(A)
  Subsystem2/1(Out1) -> Sum1/1
  Subsystem/1(Out1) -> Sum1/2
  Sum1/1 -> C/1
  B/1 -> Subsystem/2(B), Subsystem2/2(B)

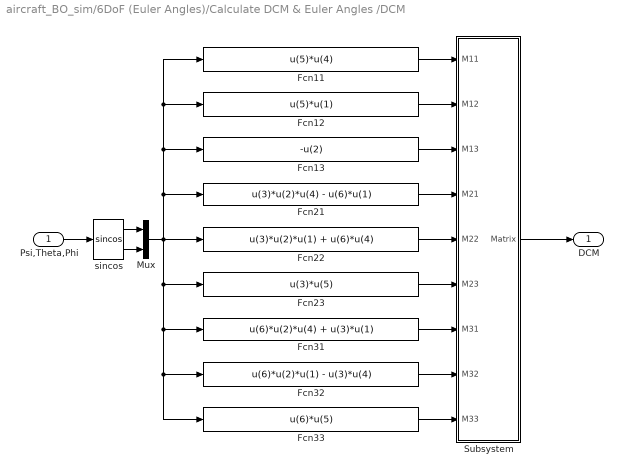
== system aircraft_BO_sim/6DoF (Euler Angles)/Calculate DCM & Euler Angles /DCM ==
  Psi,Theta,Phi : Inport  PortDimensions=3
  Fcn11 : Fcn  Expr=u(5)*u(4)
  Fcn12 : Fcn  Expr=u(5)*u(1)
  Fcn13 : Fcn  Expr=-u(2)
  Fcn21 : Fcn  Expr=u(3)*u(2)*u(4) - u(6)*u(1)
  Fcn22 : Fcn  Expr=u(3)*u(2)*u(1) + u(6)*u(4)
  Fcn23 : Fcn  Expr=u(3)*u(5)
  Fcn31 : Fcn  Expr=u(6)*u(2)*u(4) + u(3)*u(1)
  Fcn32 : Fcn  Expr=u(6)*u(2)*u(1) - u(3)*u(4)
  Fcn33 : Fcn  Expr=u(6)*u(5)
  Mux : Mux  Inputs=2
  Subsystem : Subsystem
  sincos : Trigonometry  Operator=sincos
  DCM : Outport  PortDimensions=[3,3]
  wires:
  Fcn11/1 -> Subsystem/1(M11)
  Fcn12/1 -> Subsystem/2(M12)
  Fcn13/1 -> Subsystem/3(M13)
  Fcn21/1 -> Subsystem/4(M21)
  Fcn31/1 -> Subsystem/7(M31)
  Fcn22/1 -> Subsystem/5(M22)
  Fcn23/1 -> Subsystem/6(M23)
  Fcn32/1 -> Subsystem/8(M32)
  Fcn33/1 -> Subsystem/9(M33)
  Psi,Theta,Phi/1 -> sincos/1
  Subsystem/1(Matrix) -> DCM/1
  sincos/1 -> Mux/1
  sincos/2 -> Mux/2
  Mux/1 -> Fcn11/1, Fcn12/1, Fcn13/1, Fcn21/1, Fcn32/1, Fcn33/1, Fcn31/1, Fcn23/1, Fcn22/1

== system aircraft_BO_sim/6DoF (Euler Angles)/Calculate DCM & Euler Angles /Subsystem ==
  p q r : Inport
  phi theta psi : Inport  Port=2
  Mux1 : Mux  Inputs=[3 3 3]
  Mux2 : Mux  Inputs=3
  phidot : Fcn  Expr=u[1]+(u[2]*u[4]+u[3]*u[7])*(u[5]/u[8])
  psidot : Fcn  Expr=(u[2]*u[4]+u[3]*u[7])/u[8]
  sincos : Trigonometry  Operator=sincos
  thetadot : Fcn  Expr=u[2]*u[7]-u[3]*u[4]
  phidot thetadot psidot : Outport
  wires:
  Mux1/1 -> psidot/1, phidot/1, thetadot/1
  p q r/1 -> Mux1/1
  phi theta psi/1 -> sincos/1
  psidot/1 -> Mux2/3
  thetadot/1 -> Mux2/2
  phidot/1 -> Mux2/1
  Mux2/1 -> phidot thetadot psidot/1
  sincos/1 -> Mux1/2
  sincos/2 -> Mux1/3

== system aircraft_BO_sim/6DoF (Euler Angles)/Cross Product/Subsystem ==
  A : Inport
  B : Inport  Port=2
  Demux : Demux  Outputs=3
  Demux1 : Demux  Outputs=3
  Mux : Mux  Inputs=3
  i x k : Product  InputSameDT=on  SaturateOnIntegerOverflow=on  OutDataTypeStr=Inherit: Same as first input
  j x i : Product  InputSameDT=on  SaturateOnIntegerOverflow=on  OutDataTypeStr=Inherit: Same as first input
  k x j : Product  InputSameDT=on  SaturateOnIntegerOverflow=on  OutDataTypeStr=Inherit: Same as first input
  Out1 : Outport
  wires:
  j x i/1 -> Mux/3
  i x k/1 -> Mux/2
  k x j/1 -> Mux/1
  Mux/1 -> Out1/1
  Demux1/1 -> j x i/2
  Demux/2 -> j x i/1
  Demux1/3 -> i x k/2
  Demux/1 -> i x k/1
  Demux1/2 -> k x j/2
  Demux/3 -> k x j/1
  B/1 -> Demux1/1
  A/1 -> Demux/1

== system aircraft_BO_sim/6DoF (Euler Angles)/Cross Product/Subsystem2 ==
  A : Inport
  B : Inport  Port=2
  Demux : Demux  Outputs=3
  Demux1 : Demux  Outputs=3
  Mux : Mux  Inputs=3
  i x j : Product  InputSameDT=on  SaturateOnIntegerOverflow=on  OutDataTypeStr=Inherit: Same as first input
  j x k : Product  InputSameDT=on  SaturateOnIntegerOverflow=on  OutDataTypeStr=Inherit: Same as first input
  k x i : Product  InputSameDT=on  SaturateOnIntegerOverflow=on  OutDataTypeStr=Inherit: Same as first input
  Out1 : Outport
  wires:
  Demux/3 -> k x i/1
  Demux1/2 -> i x j/2
  k x i/1 -> Mux/2
  i x j/1 -> Mux/3
  Demux/1 -> i x j/1
  Demux1/1 -> k x i/2
  Demux1/3 -> j x k/2
  Mux/1 -> Out1/1
  j x k/1 -> Mux/1
  B/1 -> Demux1/1
  A/1 -> Demux/1
  Demux/2 -> j x k/1

== system aircraft_BO_sim/6DoF (Euler Angles)/omega_dot/Cross Product ==
  A : Inport
  B : Inport  Port=2
  Subsystem : Subsystem
  Subsystem2 : Subsystem
  Sum1 : Sum  Inputs=+|-  InputSameDT=on  SaturateOnIntegerOverflow=on  OutDataTypeStr=Inherit: Same as first input
  C : Outport
  wires:
  A/1 -> Subsystem/1(A), Subsystem2/1(A)
  Subsystem2/1(Out1) -> Sum1/1
  Subsystem/1(Out1) -> Sum1/2
  Sum1/1 -> C/1
  B/1 -> Subsystem/2(B), Subsystem2/2(B)

== system aircraft_BO_sim/6DoF (Euler Angles)/omega_dot/Subsystem1 ==
  p q r : Inport
  Inertia : Inport  Port=2
  Product : Product  Multiplication=Matrix(*)  InputSameDT=on  SaturateOnIntegerOverflow=on  OutDataTypeStr=Inherit: Same as first input
  Reshape2 : Reshape  OutputDimensionality=Column vector (2-D)
  Reshape3 : Reshape
  I * w : Outport
  wires:
  Inertia/1 -> Product/1
  p q r/1 -> Reshape2/1
  Product/1 -> Reshape3/1
  Reshape3/1 -> I * w/1
  Reshape2/1 -> Product/2

== system aircraft_BO_sim/Propulsion/Cross Product/Subsystem ==
  A : Inport
  B : Inport  Port=2
  Demux : Demux  Outputs=3
  Demux1 : Demux  Outputs=3
  Mux : Mux  Inputs=3
  i x k : Product  InputSameDT=on  SaturateOnIntegerOverflow=on  OutDataTypeStr=Inherit: Same as first input
  j x i : Product  InputSameDT=on  SaturateOnIntegerOverflow=on  OutDataTypeStr=Inherit: Same as first input
  k x j : Product  InputSameDT=on  SaturateOnIntegerOverflow=on  OutDataTypeStr=Inherit: Same as first input
  Out1 : Outport
  wires:
  j x i/1 -> Mux/3
  i x k/1 -> Mux/2
  k x j/1 -> Mux/1
  Mux/1 -> Out1/1
  Demux1/1 -> j x i/2
  Demux/2 -> j x i/1
  Demux1/3 -> i x k/2
  Demux/1 -> i x k/1
  Demux1/2 -> k x j/2
  Demux/3 -> k x j/1
  B/1 -> Demux1/1
  A/1 -> Demux/1

== system aircraft_BO_sim/Propulsion/Cross Product/Subsystem2 ==
  A : Inport
  B : Inport  Port=2
  Demux : Demux  Outputs=3
  Demux1 : Demux  Outputs=3
  Mux : Mux  Inputs=3
  i x j : Product  InputSameDT=on  SaturateOnIntegerOverflow=on  OutDataTypeStr=Inherit: Same as first input
  j x k : Product  InputSameDT=on  SaturateOnIntegerOverflow=on  OutDataTypeStr=Inherit: Same as first input
  k x i : Product  InputSameDT=on  SaturateOnIntegerOverflow=on  OutDataTypeStr=Inherit: Same as first input
  Out1 : Outport
  wires:
  Demux/3 -> k x i/1
  Demux1/2 -> i x j/2
  k x i/1 -> Mux/2
  i x j/1 -> Mux/3
  Demux/1 -> i x j/1
  Demux1/1 -> k x i/2
  Demux1/3 -> j x k/2
  Mux/1 -> Out1/1
  j x k/1 -> Mux/1
  B/1 -> Demux1/1
  A/1 -> Demux/1
  Demux/2 -> j x k/1

== system aircraft_BO_sim/Propulsion/Cross Product1/Subsystem ==
  A : Inport
  B : Inport  Port=2
  Demux : Demux  Outputs=3
  Demux1 : Demux  Outputs=3
  Mux : Mux  Inputs=3
  i x k : Product  InputSameDT=on  SaturateOnIntegerOverflow=on  OutDataTypeStr=Inherit: Same as first input
  j x i : Product  InputSameDT=on  SaturateOnIntegerOverflow=on  OutDataTypeStr=Inherit: Same as first input
  k x j : Product  InputSameDT=on  SaturateOnIntegerOverflow=on  OutDataTypeStr=Inherit: Same as first input
  Out1 : Outport
  wires:
  j x i/1 -> Mux/3
  i x k/1 -> Mux/2
  k x j/1 -> Mux/1
  Mux/1 -> Out1/1
  Demux1/1 -> j x i/2
  Demux/2 -> j x i/1
  Demux1/3 -> i x k/2
  Demux/1 -> i x k/1
  Demux1/2 -> k x j/2
  Demux/3 -> k x j/1
  B/1 -> Demux1/1
  A/1 -> Demux/1

== system aircraft_BO_sim/Propulsion/Cross Product1/Subsystem2 ==
  A : Inport
  B : Inport  Port=2
  Demux : Demux  Outputs=3
  Demux1 : Demux  Outputs=3
  Mux : Mux  Inputs=3
  i x j : Product  InputSameDT=on  SaturateOnIntegerOverflow=on  OutDataTypeStr=Inherit: Same as first input
  j x k : Product  InputSameDT=on  SaturateOnIntegerOverflow=on  OutDataTypeStr=Inherit: Same as first input
  k x i : Product  InputSameDT=on  SaturateOnIntegerOverflow=on  OutDataTypeStr=Inherit: Same as first input
  Out1 : Outport
  wires:
  Demux/3 -> k x i/1
  Demux1/2 -> i x j/2
  k x i/1 -> Mux/2
  i x j/1 -> Mux/3
  Demux/1 -> i x j/1
  Demux1/1 -> k x i/2
  Demux1/3 -> j x k/2
  Mux/1 -> Out1/1
  j x k/1 -> Mux/1
  B/1 -> Demux1/1
  A/1 -> Demux/1
  Demux/2 -> j x k/1

== system aircraft_BO_sim/6DoF (Euler Angles)/Calculate DCM & Euler Angles /DCM/Subsystem ==
  M11 : Inport  PortDimensions=1
  M12 : Inport  Port=2  PortDimensions=1
  M13 : Inport  Port=3  PortDimensions=1
  M21 : Inport  Port=4  PortDimensions=1
  M22 : Inport  Port=5  PortDimensions=1
  M23 : Inport  Port=6  PortDimensions=1
  M31 : Inport  Port=7  PortDimensions=1
  M32 : Inport  Port=8  PortDimensions=1
  M33 : Inport  Port=9  PortDimensions=1
  Reshape (9) to [3x3] column-major : Reshape  OutputDimensionality=Customize  OutputDimensions=[3,3]
  Vector Concatenate : Concatenate  NumInputs=9
  Matrix : Outport  PortDimensions=[3 3]
  wires:
  M32/1 -> Vector Concatenate/6
  Reshape (9) to [3x3] column-major/1 -> Matrix/1
  M22/1 -> Vector Concatenate/5
  M12/1 -> Vector Concatenate/4
  M33/1 -> Vector Concatenate/9
  M23/1 -> Vector Concatenate/8
  M13/1 -> Vector Concatenate/7
  M11/1 -> Vector Concatenate/1
  Vector Concatenate/1 -> Reshape (9) to [3x3] column-major/1
  M31/1 -> Vector Concatenate/3
  M21/1 -> Vector Concatenate/2

== system aircraft_BO_sim/6DoF (Euler Angles)/omega_dot/Cross Product/Subsystem ==
  A : Inport
  B : Inport  Port=2
  Demux : Demux  Outputs=3
  Demux1 : Demux  Outputs=3
  Mux : Mux  Inputs=3
  i x k : Product  InputSameDT=on  SaturateOnIntegerOverflow=on  OutDataTypeStr=Inherit: Same as first input
  j x i : Product  InputSameDT=on  SaturateOnIntegerOverflow=on  OutDataTypeStr=Inherit: Same as first input
  k x j : Product  InputSameDT=on  SaturateOnIntegerOverflow=on  OutDataTypeStr=Inherit: Same as first input
  Out1 : Outport
  wires:
  j x i/1 -> Mux/3
  i x k/1 -> Mux/2
  k x j/1 -> Mux/1
  Mux/1 -> Out1/1
  Demux1/1 -> j x i/2
  Demux/2 -> j x i/1
  Demux1/3 -> i x k/2
  Demux/1 -> i x k/1
  Demux1/2 -> k x j/2
  Demux/3 -> k x j/1
  B/1 -> Demux1/1
  A/1 -> Demux/1

== system aircraft_BO_sim/6DoF (Euler Angles)/omega_dot/Cross Product/Subsystem2 ==
  A : Inport
  B : Inport  Port=2
  Demux : Demux  Outputs=3
  Demux1 : Demux  Outputs=3
  Mux : Mux  Inputs=3
  i x j : Product  InputSameDT=on  SaturateOnIntegerOverflow=on  OutDataTypeStr=Inherit: Same as first input
  j x k : Product  InputSameDT=on  SaturateOnIntegerOverflow=on  OutDataTypeStr=Inherit: Same as first input
  k x i : Product  InputSameDT=on  SaturateOnIntegerOverflow=on  OutDataTypeStr=Inherit: Same as first input
  Out1 : Outport
  wires:
  Demux/3 -> k x i/1
  Demux1/2 -> i x j/2
  k x i/1 -> Mux/2
  i x j/1 -> Mux/3
  Demux/1 -> i x j/1
  Demux1/1 -> k x i/2
  Demux1/3 -> j x k/2
  Mux/1 -> Out1/1
  j x k/1 -> Mux/1
  B/1 -> Demux1/1
  A/1 -> Demux/1
  Demux/2 -> j x k/1
